simulink model "Discrete_Time_Sim_With_Noise"  (R2024b)
settings: Solver=FixedStepAuto  StartTime=0.0  StopTime=10  FixedStep=0.001  RelTol=1e-3
undefined symbols (not defined in the file or in its folder): DiscIntNeverNeededParam, dspblkCoreblockFVToolHelper, gcbh
libraries: simulink x12, sharedTrackingLibrary x1
(part 2 of 4)

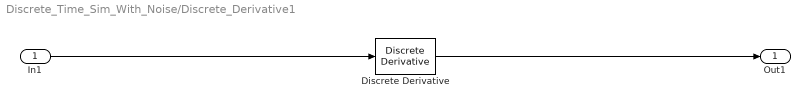
== system Discrete_Time_Sim_With_Noise/Discrete_Derivative1 ==
  In1 : Inport
  Discrete Derivative : simulink/Discrete/Discrete Derivative  gainval=1.0  ICPrevScaledInput=0.0  InputProcessing=Columns as channels (frame based)  OutMin=[]  OutMax=[]  OutDataType=fixdt(1, 16)  OutScaling=2^-10  DoSatur=off
  Out1 : Outport
  wires:
  In1/1 -> Discrete Derivative/1
  Discrete Derivative/1 -> Out1/1

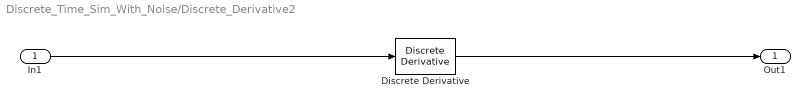
== system Discrete_Time_Sim_With_Noise/Discrete_Derivative2 ==
  In1 : Inport
  Discrete Derivative : simulink/Discrete/Discrete Derivative  gainval=1.0  ICPrevScaledInput=0.0  InputProcessing=Columns as channels (frame based)  OutMin=[]  OutMax=[]  OutDataType=fixdt(1, 16)  OutScaling=2^-10  DoSatur=off
  Out1 : Outport
  wires:
  In1/1 -> Discrete Derivative/1
  Discrete Derivative/1 -> Out1/1

== system Discrete_Time_Sim_With_Noise/Discrete_Derivative3 ==
  In1 : Inport
  Discrete Derivative : simulink/Discrete/Discrete Derivative  gainval=1.0  ICPrevScaledInput=0.0  InputProcessing=Columns as channels (frame based)  OutMin=[]  OutMax=[]  OutDataType=fixdt(1, 16)  OutScaling=2^-10  DoSatur=off
  Out1 : Outport
  wires:
  In1/1 -> Discrete Derivative/1
  Discrete Derivative/1 -> Out1/1

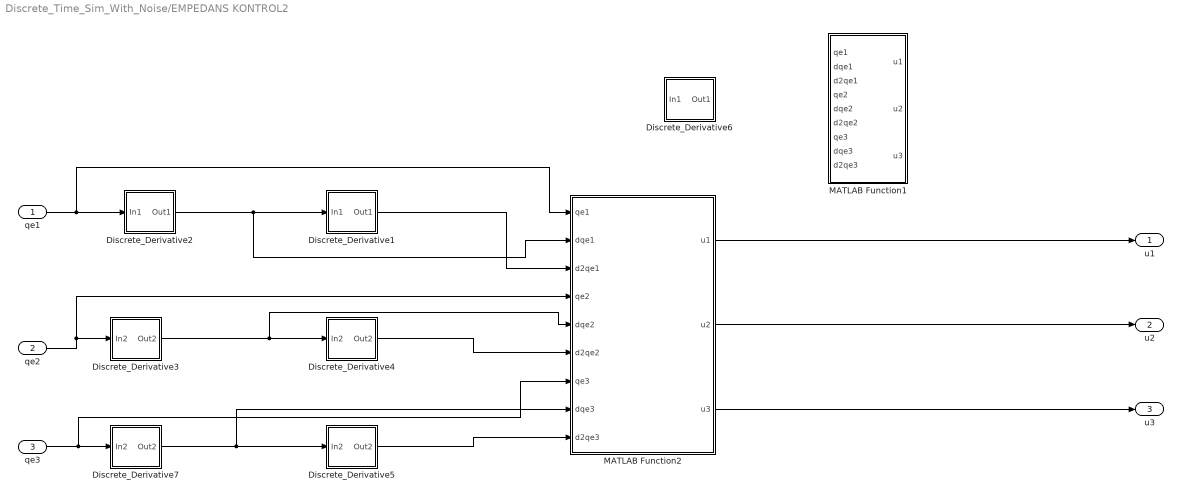
== system Discrete_Time_Sim_With_Noise/EMPEDANS KONTROL2 ==
  qe1 : Inport
  qe2 : Inport  Port=2
  qe3 : Inport  Port=3
  Discrete_Derivative1 : Subsystem
  Discrete_Derivative2 : Subsystem
  Discrete_Derivative3 : Subsystem
  Discrete_Derivative4 : Subsystem
  Discrete_Derivative5 : Subsystem
  Discrete_Derivative6 : Subsystem
  Discrete_Derivative7 : Subsystem
  MATLAB Function1 : MATLAB Function  TreatAsAtomicUnit=on
  MATLAB Function2 : MATLAB Function  TreatAsAtomicUnit=on
  u1 : Outport
  u2 : Outport  Port=2
  u3 : Outport  Port=3
  wires:
  qe1/1 -> Discrete_Derivative2/1(In1), MATLAB Function2/1(qe1)
  qe2/1 -> Discrete_Derivative3/1(In2), MATLAB Function2/4(qe2)
  qe3/1 -> MATLAB Function2/7(qe3), Discrete_Derivative7/1(In2)
  Discrete_Derivative2/1(Out1) -> MATLAB Function2/2(dqe1), Discrete_Derivative1/1(In1)
  Discrete_Derivative3/1(Out2) -> Discrete_Derivative4/1(In2), MATLAB Function2/5(dqe2)
  Discrete_Derivative7/1(Out2) -> MATLAB Function2/8(dqe3), Discrete_Derivative5/1(In2)
  Discrete_Derivative1/1(Out1) -> MATLAB Function2/3(d2qe1)
  Discrete_Derivative4/1(Out2) -> MATLAB Function2/6(d2qe2)
  Discrete_Derivative5/1(Out2) -> MATLAB Function2/9(d2qe3)
  MATLAB Function2/1(u1) -> u1/1
  MATLAB Function2/2(u2) -> u2/1
  MATLAB Function2/3(u3) -> u3/1

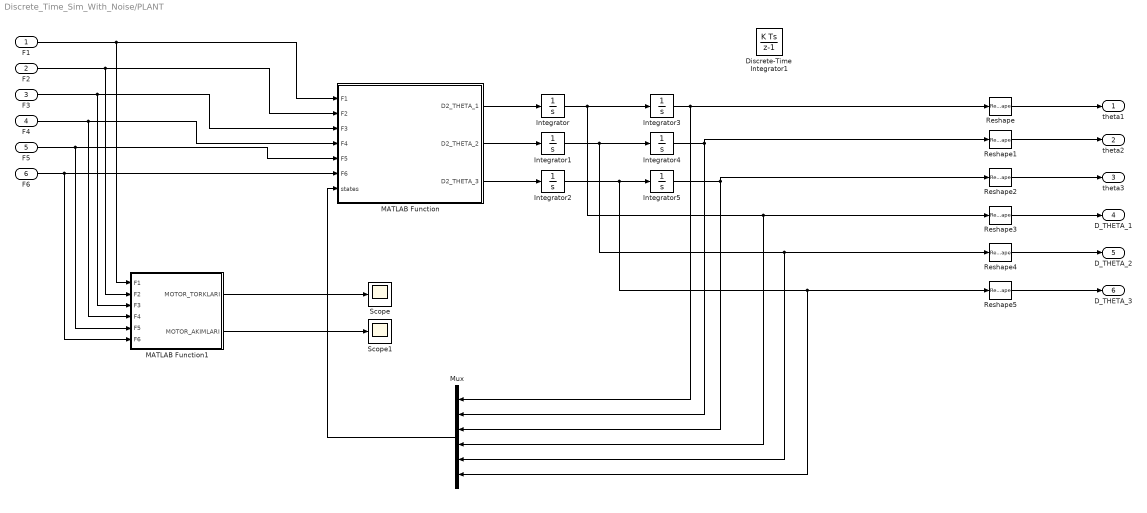
== system Discrete_Time_Sim_With_Noise/PLANT ==
  F1 : Inport
  F2 : Inport  Port=2
  F3 : Inport  Port=3
  F4 : Inport  Port=4
  F5 : Inport  Port=5
  F6 : Inport  Port=6
  Discrete-Time Integrator1 : DiscreteIntegrator  SampleTime=0.001  ICPrevOutput=DiscIntNeverNeededParam  ICPrevScaledInput=DiscIntNeverNeededParam
  Integrator{,1..5} (6 alike) : Integrator
  MATLAB Function : MATLAB Function  TreatAsAtomicUnit=on
  MATLAB Function1 : MATLAB Function  TreatAsAtomicUnit=on
  Mux : Mux  Inputs=6
  Reshape{,1..5} (6 alike) : Reshape  OutputDimensionality=Customize
  Scope : Scope
  Scope1 : Scope
  theta1 : Outport
  theta2 : Outport  Port=2
  theta3 : Outport  Port=3
  D_THETA_1 : Outport  Port=4
  D_THETA_2 : Outport  Port=5
  D_THETA_3 : Outport  Port=6
  wires:
  MATLAB Function/1(D2_THETA_1) -> Integrator/1
  MATLAB Function/2(D2_THETA_2) -> Integrator1/1
  MATLAB Function/3(D2_THETA_3) -> Integrator2/1
  Integrator/1 -> Integrator3/1, Mux/4, Reshape3/1
  Integrator1/1 -> Integrator4/1, Mux/5, Reshape4/1
  Integrator2/1 -> Integrator5/1, Mux/6, Reshape5/1
  Integrator4/1 -> Reshape1/1, Mux/2
  Integrator5/1 -> Reshape2/1, Mux/3
  F1/1 -> MATLAB Function1/1(F1), MATLAB Function/1(F1)
  F2/1 -> MATLAB Function/2(F2), MATLAB Function1/2(F2)
  F3/1 -> MATLAB Function/3(F3), MATLAB Function1/3(F3)
  F4/1 -> MATLAB Function/4(F4), MATLAB Function1/4(F4)
  Mux/1 -> MATLAB Function/7(states)
  Integrator3/1 -> Reshape/1, Mux/1
  F5/1 -> MATLAB Function/5(F5), MATLAB Function1/5(F5)
  F6/1 -> MATLAB Function/6(F6), MATLAB Function1/6(F6)
  MATLAB Function1/1(MOTOR_TORKLARI) -> Scope/1
  MATLAB Function1/2(MOTOR_AKIMLARI) -> Scope1/1
  Reshape/1 -> theta1/1
  Reshape1/1 -> theta2/1
  Reshape2/1 -> theta3/1
  Reshape3/1 -> D_THETA_1/1
  Reshape4/1 -> D_THETA_2/1
  Reshape5/1 -> D_THETA_3/1

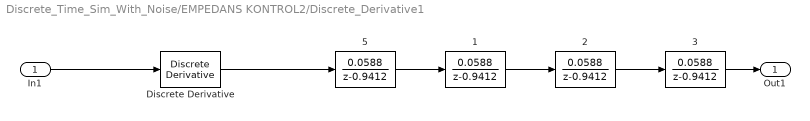
== system Discrete_Time_Sim_With_Noise/EMPEDANS KONTROL2/Discrete_Derivative1 ==
  In1 : Inport
  {1..3,5} (4 alike) : DiscreteTransferFcn  LoadFcn=dspblkCoreblockFVToolHelper(gcbh,'load');  Numerator=[0.0588]  Denominator=[1 -0.9412]
      settings: CopyFcn=dspblkCoreblockFVToolHelper(gcbh,'copy');  DeleteFcn=dspblkCoreblockFVToolHelper(gcbh,'close');  ModelCloseFcn=dspblkCoreblockFVToolHelper(gcbh,'close');  PreSaveFcn=dspblkCoreblockFVToolHelper(gcbh,'presave');  PostSaveFcn=dspblkCoreblockFVToolHelper(gcbh,'postsave');  CloseFcn=dspblkCoreblockFVToolHelper(gcbh,'close');
  Discrete Derivative : simulink/Discrete/Discrete Derivative  gainval=1.0  ICPrevScaledInput=0.0  InputProcessing=Columns as channels (frame based)  OutMin=[]  OutMax=[]  OutDataType=fixdt(1, 16)  OutScaling=2^-10  DoSatur=off
  Out1 : Outport
  wires:
  Discrete Derivative/1 -> 5/1
  5/1 -> 1/1
  1/1 -> 2/1
  In1/1 -> Discrete Derivative/1
  2/1 -> 3/1
  3/1 -> Out1/1

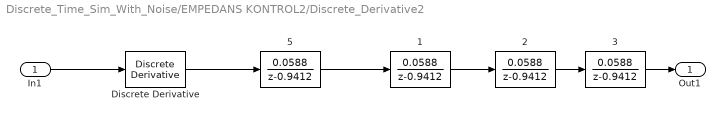
== system Discrete_Time_Sim_With_Noise/EMPEDANS KONTROL2/Discrete_Derivative2 ==
  In1 : Inport
  {1..3,5} (4 alike) : DiscreteTransferFcn  LoadFcn=dspblkCoreblockFVToolHelper(gcbh,'load');  Numerator=[0.0588]  Denominator=[1 -0.9412]
      settings: CopyFcn=dspblkCoreblockFVToolHelper(gcbh,'copy');  DeleteFcn=dspblkCoreblockFVToolHelper(gcbh,'close');  ModelCloseFcn=dspblkCoreblockFVToolHelper(gcbh,'close');  PreSaveFcn=dspblkCoreblockFVToolHelper(gcbh,'presave');  PostSaveFcn=dspblkCoreblockFVToolHelper(gcbh,'postsave');  CloseFcn=dspblkCoreblockFVToolHelper(gcbh,'close');
  Discrete Derivative : simulink/Discrete/Discrete Derivative  gainval=1.0  ICPrevScaledInput=0.0  InputProcessing=Columns as channels (frame based)  OutMin=[]  OutMax=[]  OutDataType=fixdt(1, 16)  OutScaling=2^-10  DoSatur=off
  Out1 : Outport
  wires:
  Discrete Derivative/1 -> 5/1
  In1/1 -> Discrete Derivative/1
  5/1 -> 1/1
  1/1 -> 2/1
  2/1 -> 3/1
  3/1 -> Out1/1

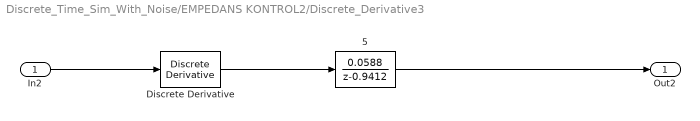
== system Discrete_Time_Sim_With_Noise/EMPEDANS KONTROL2/Discrete_Derivative3 ==
  In2 : Inport
  5 : DiscreteTransferFcn  LoadFcn=dspblkCoreblockFVToolHelper(gcbh,'load');  Numerator=[0.0588]  Denominator=[1 -0.9412]
      settings: CopyFcn=dspblkCoreblockFVToolHelper(gcbh,'copy');  DeleteFcn=dspblkCoreblockFVToolHelper(gcbh,'close');  ModelCloseFcn=dspblkCoreblockFVToolHelper(gcbh,'close');  PreSaveFcn=dspblkCoreblockFVToolHelper(gcbh,'presave');  PostSaveFcn=dspblkCoreblockFVToolHelper(gcbh,'postsave');  CloseFcn=dspblkCoreblockFVToolHelper(gcbh,'close');
  Discrete Derivative : simulink/Discrete/Discrete Derivative  gainval=1.0  ICPrevScaledInput=0.0  InputProcessing=Columns as channels (frame based)  OutMin=[]  OutMax=[]  OutDataType=fixdt(1, 16)  OutScaling=2^-10  DoSatur=off
  Out2 : Outport
  wires:
  In2/1 -> Discrete Derivative/1
  Discrete Derivative/1 -> 5/1
  5/1 -> Out2/1

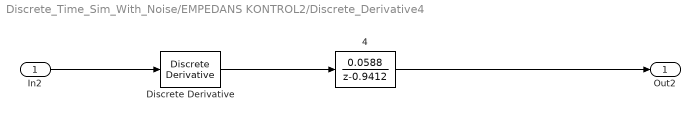
== system Discrete_Time_Sim_With_Noise/EMPEDANS KONTROL2/Discrete_Derivative4 ==
  In2 : Inport
  4 : DiscreteTransferFcn  LoadFcn=dspblkCoreblockFVToolHelper(gcbh,'load');  Numerator=[0.0588]  Denominator=[1 -0.9412]
      settings: CopyFcn=dspblkCoreblockFVToolHelper(gcbh,'copy');  DeleteFcn=dspblkCoreblockFVToolHelper(gcbh,'close');  ModelCloseFcn=dspblkCoreblockFVToolHelper(gcbh,'close');  PreSaveFcn=dspblkCoreblockFVToolHelper(gcbh,'presave');  PostSaveFcn=dspblkCoreblockFVToolHelper(gcbh,'postsave');  CloseFcn=dspblkCoreblockFVToolHelper(gcbh,'close');
  Discrete Derivative : simulink/Discrete/Discrete Derivative  gainval=1.0  ICPrevScaledInput=0.0  InputProcessing=Columns as channels (frame based)  OutMin=[]  OutMax=[]  OutDataType=fixdt(1, 16)  OutScaling=2^-10  DoSatur=off
  Out2 : Outport
  wires:
  4/1 -> Out2/1
  Discrete Derivative/1 -> 4/1
  In2/1 -> Discrete Derivative/1

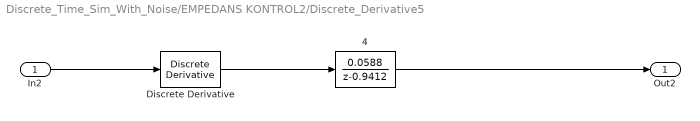
== system Discrete_Time_Sim_With_Noise/EMPEDANS KONTROL2/Discrete_Derivative5 ==
  In2 : Inport
  4 : DiscreteTransferFcn  LoadFcn=dspblkCoreblockFVToolHelper(gcbh,'load');  Numerator=[0.0588]  Denominator=[1 -0.9412]
      settings: CopyFcn=dspblkCoreblockFVToolHelper(gcbh,'copy');  DeleteFcn=dspblkCoreblockFVToolHelper(gcbh,'close');  ModelCloseFcn=dspblkCoreblockFVToolHelper(gcbh,'close');  PreSaveFcn=dspblkCoreblockFVToolHelper(gcbh,'presave');  PostSaveFcn=dspblkCoreblockFVToolHelper(gcbh,'postsave');  CloseFcn=dspblkCoreblockFVToolHelper(gcbh,'close');
  Discrete Derivative : simulink/Discrete/Discrete Derivative  gainval=1.0  ICPrevScaledInput=0.0  InputProcessing=Columns as channels (frame based)  OutMin=[]  OutMax=[]  OutDataType=fixdt(1, 16)  OutScaling=2^-10  DoSatur=off
  Out2 : Outport
  wires:
  Discrete Derivative/1 -> 4/1
  In2/1 -> Discrete Derivative/1
  4/1 -> Out2/1

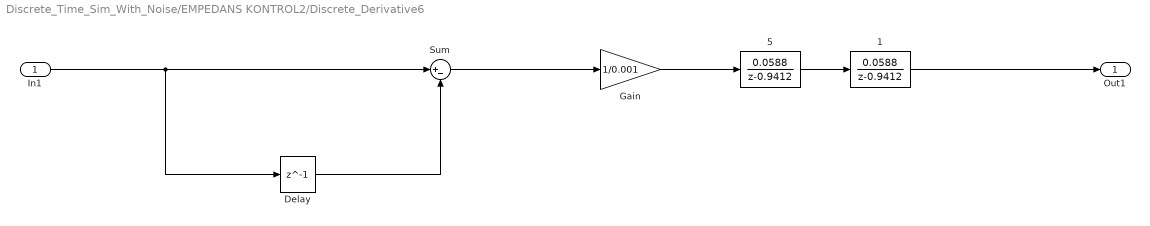
== system Discrete_Time_Sim_With_Noise/EMPEDANS KONTROL2/Discrete_Derivative6 ==
  In1 : Inport
  1 : DiscreteTransferFcn  LoadFcn=dspblkCoreblockFVToolHelper(gcbh,'load');  Numerator=[0.0588]  Denominator=[1 -0.9412]
      settings: CopyFcn=dspblkCoreblockFVToolHelper(gcbh,'copy');  DeleteFcn=dspblkCoreblockFVToolHelper(gcbh,'close');  ModelCloseFcn=dspblkCoreblockFVToolHelper(gcbh,'close');  PreSaveFcn=dspblkCoreblockFVToolHelper(gcbh,'presave');  PostSaveFcn=dspblkCoreblockFVToolHelper(gcbh,'postsave');  CloseFcn=dspblkCoreblockFVToolHelper(gcbh,'close');
  5 : DiscreteTransferFcn  LoadFcn=dspblkCoreblockFVToolHelper(gcbh,'load');  Numerator=[0.0588]  Denominator=[1 -0.9412]
      settings: CopyFcn=dspblkCoreblockFVToolHelper(gcbh,'copy');  DeleteFcn=dspblkCoreblockFVToolHelper(gcbh,'close');  ModelCloseFcn=dspblkCoreblockFVToolHelper(gcbh,'close');  PreSaveFcn=dspblkCoreblockFVToolHelper(gcbh,'presave');  PostSaveFcn=dspblkCoreblockFVToolHelper(gcbh,'postsave');  CloseFcn=dspblkCoreblockFVToolHelper(gcbh,'close');
  Delay : Delay  DelayLength=1  InputProcessing=Columns as channels (frame based)  SampleTime=0.001
  Gain : Gain  Gain=1/0.001
  Sum : Sum  Inputs=|+-
  Out1 : Outport
  wires:
  In1/1 -> Sum/1, Delay/1
  Delay/1 -> Sum/2
  Sum/1 -> Gain/1
  Gain/1 -> 5/1
  5/1 -> 1/1
  1/1 -> Out1/1

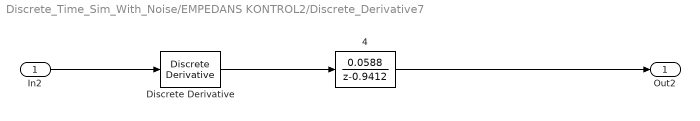
== system Discrete_Time_Sim_With_Noise/EMPEDANS KONTROL2/Discrete_Derivative7 ==
  In2 : Inport
  4 : DiscreteTransferFcn  LoadFcn=dspblkCoreblockFVToolHelper(gcbh,'load');  Numerator=[0.0588]  Denominator=[1 -0.9412]
      settings: CopyFcn=dspblkCoreblockFVToolHelper(gcbh,'copy');  DeleteFcn=dspblkCoreblockFVToolHelper(gcbh,'close');  ModelCloseFcn=dspblkCoreblockFVToolHelper(gcbh,'close');  PreSaveFcn=dspblkCoreblockFVToolHelper(gcbh,'presave');  PostSaveFcn=dspblkCoreblockFVToolHelper(gcbh,'postsave');  CloseFcn=dspblkCoreblockFVToolHelper(gcbh,'close');
  Discrete Derivative : simulink/Discrete/Discrete Derivative  gainval=1.0  ICPrevScaledInput=0.0  InputProcessing=Columns as channels (frame based)  OutMin=[]  OutMax=[]  OutDataType=fixdt(1, 16)  OutScaling=2^-10  DoSatur=off
  Out2 : Outport
  wires:
  In2/1 -> Discrete Derivative/1
  Discrete Derivative/1 -> 4/1
  4/1 -> Out2/1

== matlab function Discrete_Time_Sim_With_Noise/PLANT/MATLAB Function1 ==
  data: F1 input; MOTOR_TORKLARI output; F2 input; F3 input; F4 input; F5 input; F6 input; MOTOR_AKIMLARI output
function [MOTOR_TORKLARI, MOTOR_AKIMLARI] = fcn(F1, F2, F3, F4, F5, F6)

m1t = F1*0.0125;
m2t = F2*0.0125;
m3t = F3*0.0125;

m4t = F4*0.0125;
m5t = F5*0.0125;
m6t = F6*0.0125;

MOTOR_TORKLARI = [m1t; m2t; m3t; m4t; m5t; m6t];
MOTOR_AKIMLARI = [m1t/0.87; m2t/0.87; m3t/0.87; m4t/0.87; m5t/0.87; m6t/0.87];
end
